simulink model "GridTiedInverterNew"  (R2024b)
settings: Solver=ode45  StartTime=0.0  StopTime=1  RelTol=1e-3
PreLoadFcn:
  | run('constants.m');
InitFcn:
  | run('constants.m');
values from neighbouring files (symbols this model uses):
  f_grid = 50    [constants.m]
  K_lqi = lqi(sys, Q_lqi, R)    [constants.m]
  K_lqr = lqr(sys, Q_lqr, R)    [constants.m]
  Ki = alpha * w_grid * w_grid * T_p * L_t / K_cm    (= 6152.69773705)    [constants.m]
  Ki_ = 10    [constants.m]
  Kp = (T_p * L_t * (2 * zeta * w_grid * alpha + w_grid * w_grid) - R_t) / K_cm    (= 28.1407059403)    [constants.m]
  Kp_ = 7000    [constants.m]
  L_t = 5e-2    (= 0.05)    [constants.m]
  P_rated_transformer = 10e3    (= 10000)    [constants.m]
  R_t = 0.15    [constants.m]
  t_breaker_on = 0.2    [constants.m]
  t_sample = 1 / f_sample    (= 1e-05)    [constants.m]
  V_dc = 300    [constants.m]
  V_grid = 230 * 4    (= 920)    [constants.m]
  V_t = 230    [constants.m]
undefined symbols (not defined in the file or in its folder): Kcp
libraries: spsIGBTDiodeLib x6, spsThreePhaseVIMeasurementLib x2, spsabctodq0Lib x2, spsPower3phInstantaneousLib x2, spsThreePhaseBreakerLib x1, spsThreePhaseSourceLib x1, spsPLL3phLib x1, spsThreePhaseSeriesRLCBranchLib x1, spsSawtoothGeneratorLib x1, spsTHDLib x1, SignalEditorBlockLib x1, eePwmGeneratorTwoLevel x1
settings Model: Creator=Gilbert  LastModifiedBy=Gilbert

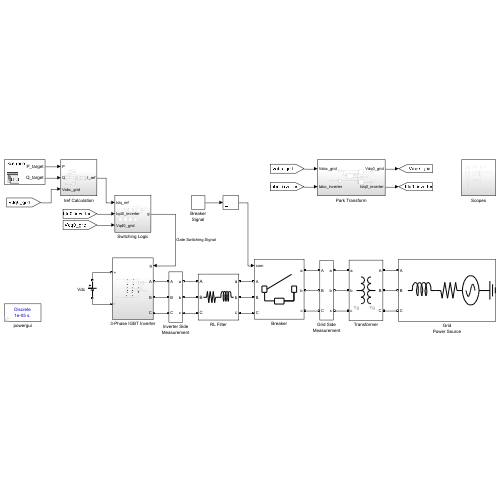
[thumbnail: Simulink's stored preview of the top-level diagram]
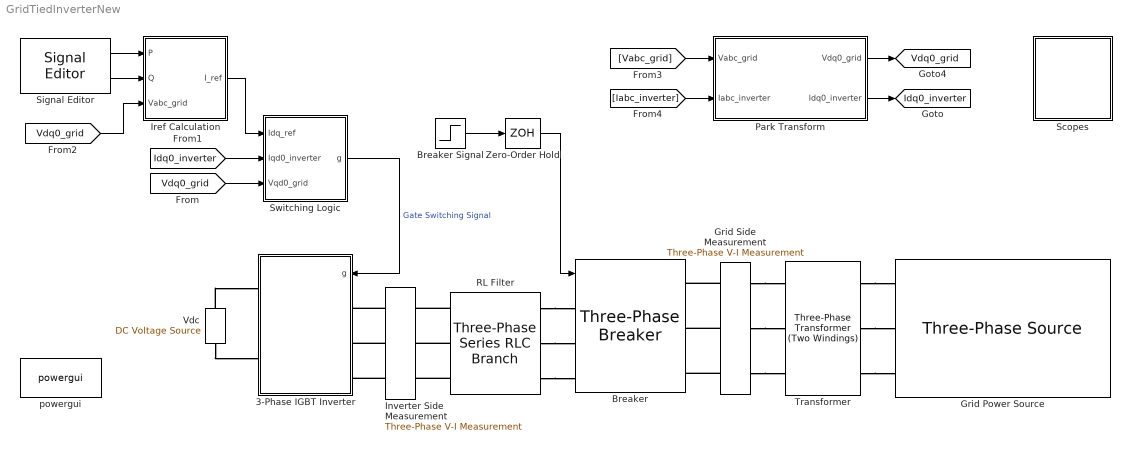
== system GridTiedInverterNew ==
  3-Phase IGBT Inverter : Subsystem
      settings: PortSchema="{\"entries\":[{\"content\":{\"sides\":[{\"content\":{\"connectorIds\":[\"LConn1\",\"LConn2\"]},\"type\":\"ConnectorPlacement.EquallySpacedRectSide\",\"uuid\":\"b894f77a-afb6-49ea-9e82-1d7302d1b564\"},{\"content\":{\"connectorIds\":[\"In1\",\"RConn1\",\"RConn2\",\"RConn3\"],\"side\":\"RIGHT\"},\"type\":\"ConnectorPlacement.EquallySpacedRectSide\",\"uuid\":\"2e0b49ec-be7c-4f2f-9d64-b0056ee6a69f\"},{\"content\":{\"side\":\"TOP\"},\"type\":\"ConnectorPlacement.EquallySpacedRectSide\",\"uuid\":\"c0a39988-5ea5-41cc-9f2f-ca3dfeeba5dd\"}]},\"type\":\"ConnectorPlacement.EquallySpacedConnector\",\"uuid\":\"873a7b17-3bf6-43e0-93b3-692e6d4c547a\"}],\"packageUris\":[\"http://schema.mathworks.com/mf0/Connector/R2020b\"],\"version\":\"1.0\"}"
  Breaker : spsThreePhaseBreakerLib/Three-Phase Breaker  InitialState=open  SwitchA=on  SwitchB=on  SwitchC=on  SwitchTimes="[1/60  5/60]"  External=on  BreakerResistance=0.01  SnubberResistance=1e6  SnubberCapacitance=inf  Measurements=None
  Breaker Signal : Step  Time=t_breaker_on  SampleTime=0
  Grid Power Source : spsThreePhaseSourceLib/Three-Phase Source  InternalConnection=Yg  VoltagePhases=off  Voltage=V_grid  PhaseAngle=phi_grid  Voltage_phases=[25e3 25e3 25e3]/sqrt(3)  PhaseAngles_phases=[0 -120 +120]  Frequency=f_grid  NonIdealSource=on  SpecifyImpedance=off  Resistance=0.8929e-12  Inductance=16.58e-12  ShortCircuitLevel=100e6  BaseVoltage=V_grid  XRratio=7  BusType=swing  Pref=10e3  Qref=0  Prefabc=[10e3, 10e3, 10e3]  Qrefabc=[0, 0, 0]  Qmin=-inf  Qmax=inf
  Grid Side Measurement : spsThreePhaseVIMeasurementLib/Three-Phase V-I Measurement  VoltageMeasurement=phase-to-phase  SetLabelV=on  LabelV=Vabc_grid  Vpu=off  VpuLL=off  CurrentMeasurement=yes  SetLabelI=on  LabelI=Iabc_grid  Ipu=off  Pbase=100e6  Vbase=500e3  OutputType=Complex  PhasorSimulation=off  PSBequivalent=0
  Inverter Side Measurement : spsThreePhaseVIMeasurementLib/Three-Phase V-I Measurement  VoltageMeasurement=phase-to-phase  SetLabelV=on  LabelV=Vabc_inverter  Vpu=off  VpuLL=off  CurrentMeasurement=yes  SetLabelI=on  LabelI=Iabc_inverter  Ipu=off  Pbase=100e6  Vbase=500e3  OutputType=Complex  PhasorSimulation=off  PSBequivalent=0
  Iref Calculation : Subsystem
  Park Transform : Subsystem
  RL Filter : spsThreePhaseSeriesRLCBranchLib/Three-Phase Series RLC Branch  LConnTagsString=A|B|C  RConnTagsString=A|B|C  BranchType=RL  Resistance=R_t  Inductance=L_t  Capacitance=1e-6  Measurements=None
  Scopes : Subsystem
  Signal Editor : SignalEditorBlockLib/Signal Editor  FileName=S_target_0.mat  ActiveScenario=Scenario  ActiveSignal=P_target  IsBus=off  OutputBusObjectStr=Bus: BusObject  SampleTime=0  Interpolate=off  ZeroCross=off  OutputAfterFinalValue=Holding final value  Unit=inherit  PreserveSignalName=on  ApplySigPropsToAllScenarios=on  ApplySigPropsToAllSignals=off
  Switching Logic : Subsystem
  Transformer : spsThreePhaseTransformerTwoWindingsLib/Three-Phase Transformer (Two Windings)  Winding1Connection=Yg  Winding2Connection=Yg  CoreType=Three single-phase transformers  SetSaturation=off  Hysteresis=off  DataFile='hysteresis'  SetInitialFlux=off  Measurements=None  UNITS=SI  NominalPower=[ P_rated_transformer , f_grid ]  Winding1=[V_grid 6.7712e-06 8.6214e-07]  Winding2=[V_t 4.232e-07 5.3883e-08]  Rm=1.6928  Lm=0.0053883  L0=5.3883e-06  Saturation=[0 0;532.5 2.8693;2.2187e+05 3.6344]  InitialFluxes=[1.9129 -1.9129 1.6737]  BreakLoop=off  DiscreteSolver=Trapezoidal iterative  DataType=on  TransfoNumber=1
  Vdc : spsDCVoltageSourceLib/DC Voltage Source  Amplitude=V_dc  Measurements=None
  Zero-Order Hold : ZeroOrderHold  SampleTime=t_sample
  powergui : sps_lib/powergui  Priority=1  SimulationMode=Discrete  SampleTime=t_sample  frequency=60  Iterations=50  frequencyindice=0  Pbase=100e6  ErrMax=1e-4  UnitsV=kV  UnitsW=MW  buscounter=0  FunctionMessages=off  echomessages=off  EnableUseOfTLC=off  CurrentSourceSwitches=off  DisableSnubberDevices=off  DisableRonSwitches=off  DisableVfSwitches=off  DisplayEquations=off  AutomaticDiscreteSolvers=off  SolverType=Tustin/Backward Euler (TBE)  Interpol=off  ExternalGateDelay=off  methode=off  Ts=100  x0status=blocks  SPID=on  SwTol=0  HookPort=off  NonlinearTolerance=1e-4  nMaxIteration=100  ContinueOnMaxIteration=off  RestoreLinks=warning  ResistiveCurrentMeasurement=off  Frange=[0:2:500]  Ylog=off  Xlog=on  ShowGrid=off  save=off  variable=ZData  structure=0  ZoomFFT=off  StartTime=0.0  cycles=1  DisplayStyle=1  fundamental=60  FreqAxis=off  MaxFrequency=1000  frequencyindicesteady=1  RmsSteady=1  display=off
  tag scope: Idq0_inverter=global, Vdq0_grid=global
  wires:
  [Vdq0_grid] -> Switching Logic/3(Vqd0_grid)
  [Vdq0_grid] -> Iref Calculation/3(Vabc_grid)
  Signal Editor/1 -> Iref Calculation/1(P)
  Signal Editor/2 -> Iref Calculation/2(Q)
  [Idq0_inverter] -> Switching Logic/2(Iqd0_inverter)
  Switching Logic/1(g) -> 3-Phase IGBT Inverter/1(g)  "Gate Switching Signal"
  Breaker Signal/1 -> Zero-Order Hold/1
  Zero-Order Hold/1 -> Breaker/1
  Iref Calculation/1(I_ref) -> Switching Logic/1(Idq_ref)
  Park Transform/2(Idq0_inverter) -> [Idq0_inverter]
  Park Transform/1(Vdq0_grid) -> [Vdq0_grid]
  [Vabc_grid] -> Park Transform/1(Vabc_grid)
  [Iabc_inverter] -> Park Transform/2(Iabc_inverter)
  connections:
  Transformer/LConn1 -- Grid Power Source/RConn1
  Transformer/LConn2 -- Grid Power Source/RConn2
  Transformer/LConn3 -- Grid Power Source/RConn3
  RL Filter/RConn1 -- Breaker/LConn1
  RL Filter/RConn2 -- Breaker/LConn2
  RL Filter/RConn3 -- Breaker/LConn3
  Grid Side Measurement/LConn1 -- Breaker/RConn1
  Grid Side Measurement/LConn2 -- Breaker/RConn2
  Grid Side Measurement/LConn3 -- Breaker/RConn3
  Vdc/LConn1 -- 3-Phase IGBT Inverter/LConn2
  Vdc/RConn1 -- 3-Phase IGBT Inverter/LConn1
  Inverter Side Measurement/LConn2 -- 3-Phase IGBT Inverter/RConn2
  Inverter Side Measurement/LConn3 -- 3-Phase IGBT Inverter/RConn3
  Inverter Side Measurement/LConn1 -- 3-Phase IGBT Inverter/RConn1
  Grid Side Measurement/RConn1 -- Transformer/RConn1
  Grid Side Measurement/RConn2 -- Transformer/RConn2
  Grid Side Measurement/RConn3 -- Transformer/RConn3
  RL Filter/LConn1 -- Inverter Side Measurement/RConn1
  RL Filter/LConn2 -- Inverter Side Measurement/RConn2
  RL Filter/LConn3 -- Inverter Side Measurement/RConn3

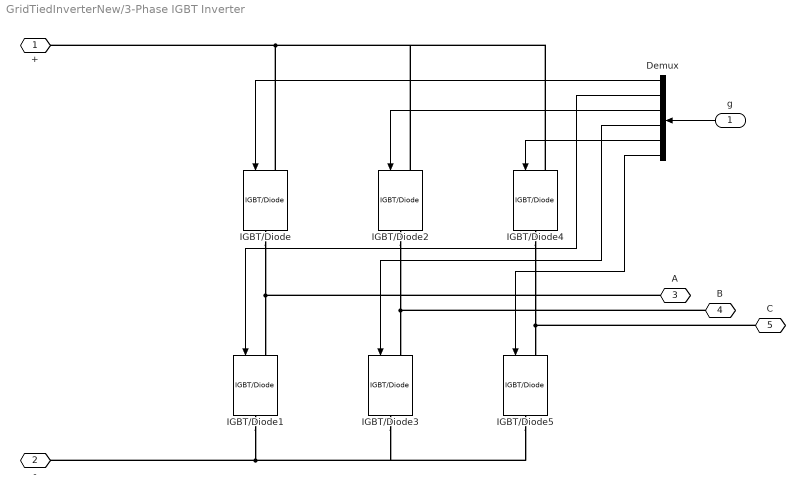
== system GridTiedInverterNew/3-Phase IGBT Inverter ==
  g : Inport
  Demux : Demux  Outputs=6
  IGBT/Diode{,1..5} (6 alike) : spsIGBTDiodeLib/IGBT//Diode  Ron=1e-3  Rs=1e5  Cs=inf  Measurements=off
  + : PMIOPort  Side=Left
  - : PMIOPort  Port=2  Side=Left
  A : PMIOPort  Port=3  Side=Right
  B : PMIOPort  Port=4  Side=Right
  C : PMIOPort  Port=5  Side=Right
  wires:
  Demux/3 -> IGBT/Diode2/1
  Demux/5 -> IGBT/Diode4/1
  Demux/2 -> IGBT/Diode1/1
  Demux/6 -> IGBT/Diode5/1
  Demux/4 -> IGBT/Diode3/1
  g/1 -> Demux/1
  Demux/1 -> IGBT/Diode/1
  connections:
  B/RConn1 -- IGBT/Diode3/LConn1 -- IGBT/Diode2/RConn1
  IGBT/Diode/LConn1 -- IGBT/Diode2/LConn1 -- IGBT/Diode4/LConn1 -- +/RConn1
  IGBT/Diode1/RConn1 -- IGBT/Diode5/RConn1 -- IGBT/Diode3/RConn1 -- -/RConn1
  A/RConn1 -- IGBT/Diode1/LConn1 -- IGBT/Diode/RConn1
  C/RConn1 -- IGBT/Diode5/LConn1 -- IGBT/Diode4/RConn1

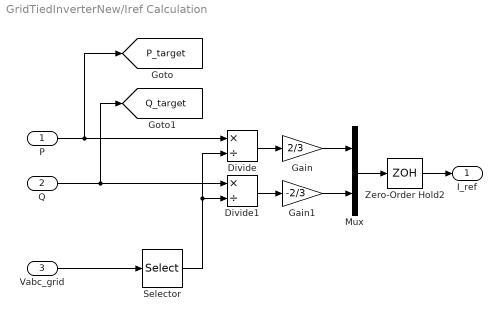
== system GridTiedInverterNew/Iref Calculation ==
  P : Inport
  Q : Inport  Port=2
  Vabc_grid : Inport  Port=3
  Divide : Product  Inputs=*/
  Divide1 : Product  Inputs=*/
  Gain : Gain  Gain=2/3
  Gain1 : Gain  Gain=-2/3
  Mux : Mux  Inputs=2
  Selector : Selector  InputPortWidth=3  IndexOptions=Index vector (dialog)  Indices=[1]  OutputSizes=1
  Zero-Order Hold2 : ZeroOrderHold  SampleTime=t_sample
  I_ref : Outport
  tag scope: P_target=global, Q_target=global
  wires:
  Vabc_grid/1 -> Selector/1
  P/1 -> [P_target], Divide/1
  Q/1 -> [Q_target], Divide1/1
  Mux/1 -> Zero-Order Hold2/1
  Selector/1 -> Divide/2, Divide1/2
  Divide/1 -> Gain/1
  Divide1/1 -> Gain1/1
  Gain/1 -> Mux/1
  Gain1/1 -> Mux/2
  Zero-Order Hold2/1 -> I_ref/1

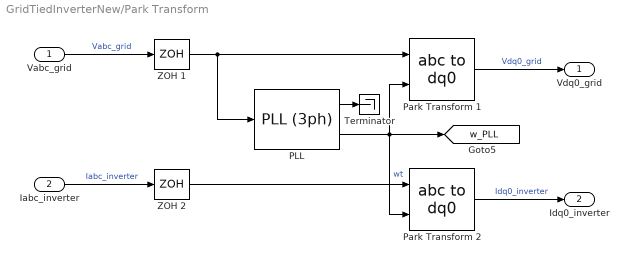
== system GridTiedInverterNew/Park Transform ==
  Vabc_grid : Inport
  Iabc_inverter : Inport  Port=2
  PLL : spsPLL3phLib/PLL (3ph)  Fmin=45  Par_Init=[0, f_grid]  ParK=[180, 3200, 1]  TcD=1e-4  MaxRateChangeFreq=12  FilterCutOffFreq=25  Ts=0  AGC=on
  Park Transform 1 : spsabctodq0Lib/abc to dq0  Alignment=90 degrees behind phase A axis
  Park Transform 2 : spsabctodq0Lib/abc to dq0  Alignment=90 degrees behind phase A axis
  Terminator : Terminator
  ZOH 1 : ZeroOrderHold  SampleTime=t_sample
  ZOH 2 : ZeroOrderHold  SampleTime=t_sample
  Vdq0_grid : Outport
  Idq0_inverter : Outport  Port=2
  tag scope: w_PLL=global
  wires:
  PLL/2 -> Park Transform 2/2, Park Transform 1/2, [w_PLL]  "wt"
  Vabc_grid/1 -> ZOH 1/1  "Vabc_grid"
  PLL/1 -> Terminator/1
  Iabc_inverter/1 -> ZOH 2/1  "Iabc_inverter"
  ZOH 1/1 -> PLL/1, Park Transform 1/1
  ZOH 2/1 -> Park Transform 2/1
  Park Transform 2/1 -> Idq0_inverter/1  "Idq0_inverter"
  Park Transform 1/1 -> Vdq0_grid/1  "Vdq0_grid"

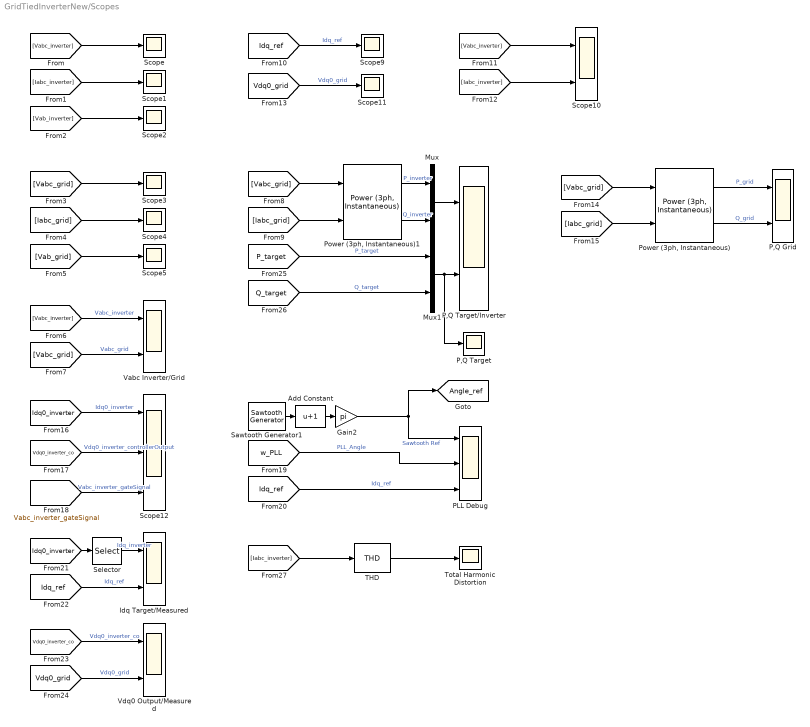
== system GridTiedInverterNew/Scopes ==
  Add Constant : Bias  Bias=1  SaturateOnIntegerOverflow=off
  Gain2 : Gain  Gain=pi
  Idq Target/Measured : Scope  NumInputPorts=2
  Mux : Mux  Inputs=2
  Mux1 : Mux  Inputs=2
  P,Q Grid : Scope  NumInputPorts=2
  P,Q Target : Scope
  P,Q Target/Inverter : Scope  NumInputPorts=2
  PLL Debug : Scope  NumInputPorts=3
  "Power (3ph, Instantaneous)" : spsPower3phInstantaneousLib/Power (3ph, Instantaneous)
  "Power (3ph, Instantaneous)1" : spsPower3phInstantaneousLib/Power (3ph, Instantaneous)
  Sawtooth Generator1 : spsSawtoothGeneratorLib/Sawtooth Generator  Freq=50  Phase=0  Ts=0
  Scope{,1..5,9,11} (8 alike) : Scope
  Scope10 : Scope  NumInputPorts=2
  Scope12 : Scope  NumInputPorts=3
  Selector : Selector  InputPortWidth=3  IndexOptions=Index vector (dialog)  Indices=[1 2]  OutputSizes=1
  THD : spsTHDLib/THD  Freq=f_grid  Ts=t_sample
  Total Harmonic Distortion : Scope
  Vabc Inverter/Grid : Scope  NumInputPorts=2
  Vdq0 Output/Measured : Scope  NumInputPorts=2
  tag scope: Angle_ref=global
  wires:
  [Vabc_inverter] -> Scope/1
  [Iabc_inverter] -> Scope1/1
  [Vab_inverter] -> Scope2/1
  [Vabc_grid] -> Scope3/1
  [Iabc_grid] -> Scope4/1
  [Vab_grid] -> Scope5/1
  [Vabc_inverter] -> Vabc Inverter/Grid/1  "Vabc_inverter"
  [Vabc_grid] -> Vabc Inverter/Grid/2  "Vabc_grid"
  [Vabc_grid] -> "Power (3ph, Instantaneous)1"/1
  [Iabc_grid] -> "Power (3ph, Instantaneous)1"/2
  "Power (3ph, Instantaneous)1"/1 -> Mux/1  "P_inverter"
  "Power (3ph, Instantaneous)1"/2 -> Mux/2  "Q_inverter"
  [Idq_ref] -> Scope9/1  "Idq_ref"
  [Vabc_inverter] -> Scope10/1
  [Iabc_inverter] -> Scope10/2
  [Vdq0_grid] -> Scope11/1  "Vdq0_grid"
  [Vabc_grid] -> "Power (3ph, Instantaneous)"/1
  [Iabc_grid] -> "Power (3ph, Instantaneous)"/2
  "Power (3ph, Instantaneous)"/1 -> P,Q Grid/1  "P_grid"
  "Power (3ph, Instantaneous)"/2 -> P,Q Grid/2  "Q_grid"
  [Idq0_inverter] -> Scope12/1  "Idq0_inverter"
  [Vdq0_inverter_co] -> Scope12/2  "Vdq0_inverter_controllerOutput"
  [Vabc_inverter_gateSignal] -> Scope12/3  "Vabc_inverter_gateSignal"
  Add Constant/1 -> Gain2/1
  Sawtooth Generator1/1 -> Add Constant/1
  [w_PLL] -> PLL Debug/2  "PLL_Angle"
  [Idq_ref] -> PLL Debug/3  "Idq_ref"
  Gain2/1 -> [Angle_ref], PLL Debug/1  "Sawtooth Ref"
  [Idq0_inverter] -> Selector/1
  [Idq_ref] -> Idq Target/Measured/2  "Idq_ref"
  [Vdq0_grid] -> Vdq0 Output/Measured/2  "Vdq0_grid"
  [Vdq0_inverter_co] -> Vdq0 Output/Measured/1  "Vdq0_inverter_co"
  [P_target] -> Mux1/1  "P_target"
  [Q_target] -> Mux1/2  "Q_target"
  Mux/1 -> P,Q Target/Inverter/1
  Mux1/1 -> P,Q Target/Inverter/2, P,Q Target/1
  [Iabc_inverter] -> THD/1
  THD/1 -> Total Harmonic Distortion/1
  Selector/1 -> Idq Target/Measured/1  "Idq_inverter"

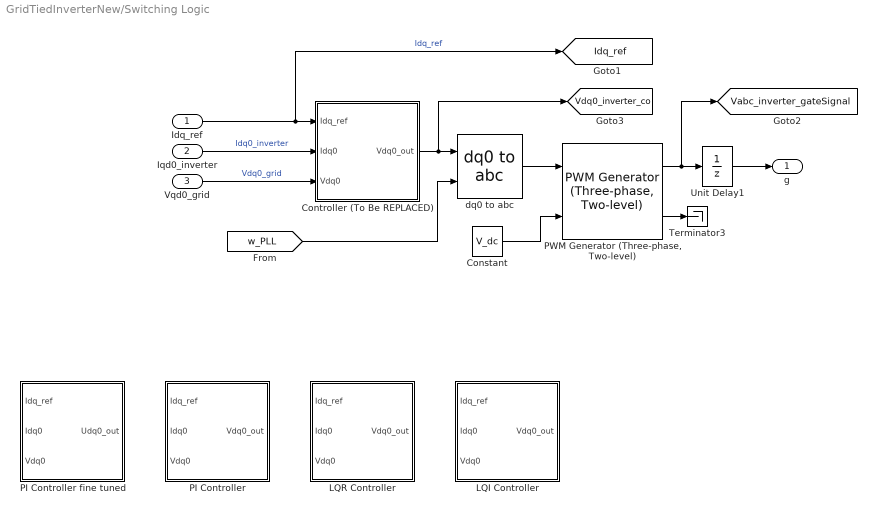
== system GridTiedInverterNew/Switching Logic ==
  Idq_ref : Inport
  Iqd0_inverter : Inport  Port=2
  Vqd0_grid : Inport  Port=3
  Constant : Constant  Value=V_dc
  Controller (To Be REPLACED) : Subsystem
  LQI Controller : Subsystem
  LQR Controller : Subsystem
  PI Controller : Subsystem
  PI Controller fine tuned : Subsystem
  "PWM Generator (Three-phase, Two-level)" : eePwmGeneratorTwoLevel/PWM Generator (Three-phase, Two-level)  PWMMode=Continuous PWM (CPWM)  CPWMMode=SVM: space vector modulation  DPWMMode=60 DPWM: 60 degree discontinuous PWM  fsw=f_sw  Ts=t_sample
      settings: LibrarySourceBlock=|
      | ee_sl_lib/Pulse Width
      | Modulation/PWM Generator
      | (Three-phase, Two-level)
  Terminator3 : Terminator
  Unit Delay1 : UnitDelay  SampleTime=t_sample  HasFrameUpgradeWarning=on
  dq0 to abc : spsdq0toabcLib/dq0 to abc  Alignment=90 degrees behind phase A axis
  g : Outport
  tag scope: Idq_ref=global, Vabc_inverter_gateSignal=global, Vdq0_inverter_co=global
  wires:
  "PWM Generator (Three-phase, Two-level)"/1 -> [Vabc_inverter_gateSignal], Unit Delay1/1
  Unit Delay1/1 -> g/1
  Constant/1 -> "PWM Generator (Three-phase, Two-level)"/2
  "PWM Generator (Three-phase, Two-level)"/2 -> Terminator3/1
  dq0 to abc/1 -> "PWM Generator (Three-phase, Two-level)"/1
  Vqd0_grid/1 -> Controller (To Be REPLACED)/3(Vdq0)  "Vdq0_grid"
  Iqd0_inverter/1 -> Controller (To Be REPLACED)/2(Idq0)  "Idq0_inverter"
  Controller (To Be REPLACED)/1(Vdq0_out) -> dq0 to abc/1, [Vdq0_inverter_co]
  Idq_ref/1 -> Controller (To Be REPLACED)/1(Idq_ref), [Idq_ref]  "Idq_ref"
  [w_PLL] -> dq0 to abc/2

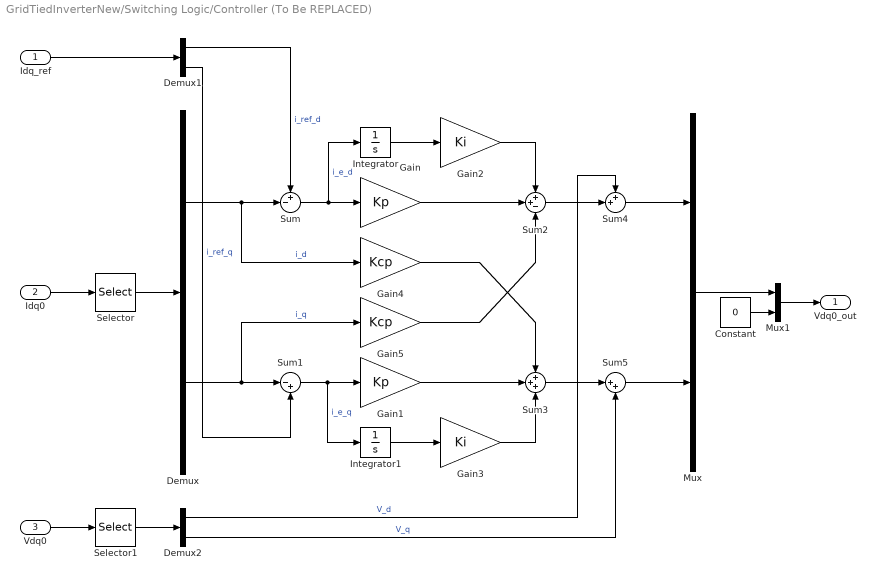
== system GridTiedInverterNew/Switching Logic/Controller (To Be REPLACED) ==
  Idq_ref : Inport
  Idq0 : Inport  Port=2
  Vdq0 : Inport  Port=3
  Constant : Constant  Value=0
  Demux : Demux  Outputs=2
  Demux1 : Demux  Outputs=2
  Demux2 : Demux  Outputs=2
  Gain : Gain  Gain=Kp
  Gain1 : Gain  Gain=Kp
  Gain2 : Gain  Gain=Ki
  Gain3 : Gain  Gain=Ki
  Gain4 : Gain  Gain=Kcp
  Gain5 : Gain  Gain=Kcp
  Integrator : Integrator
  Integrator1 : Integrator
  Mux : Mux  Inputs=2
  Mux1 : Mux  Inputs=2
  Selector : Selector  InputPortWidth=3  IndexOptions=Index vector (dialog)  Indices=[1 2]  OutputSizes=1
  Selector1 : Selector  InputPortWidth=3  IndexOptions=Index vector (dialog)  Indices=[1 2]  OutputSizes=1
  Sum : Sum  Inputs=+-|
  Sum1 : Sum  Inputs=|-+
  Sum2 : Sum  Inputs=++-
  Sum3 : Sum  Inputs=+++
  Sum4 : Sum  Inputs=++|
  Sum5 : Sum  Inputs=|++
  Vdq0_out : Outport
  wires:
  Gain5/1 -> Sum2/3
  Gain4/1 -> Sum3/1
  Demux2/2 -> Sum5/2  "V_q"
  Demux2/1 -> Sum4/1  "V_d"
  Sum5/1 -> Mux/2
  Sum3/1 -> Sum5/1
  Sum4/1 -> Mux/1
  Sum2/1 -> Sum4/2
  Selector1/1 -> Demux2/1
  Vdq0/1 -> Selector1/1
  Gain3/1 -> Sum3/3
  Integrator1/1 -> Gain3/1
  Gain1/1 -> Sum3/2
  Gain2/1 -> Sum2/1
  Integrator/1 -> Gain2/1
  Gain/1 -> Sum2/2
  Sum/1 -> Gain/1, Integrator/1  "i_e_d"
  Mux1/1 -> Vdq0_out/1
  Constant/1 -> Mux1/2
  Mux/1 -> Mux1/1
  Selector/1 -> Demux/1
  Idq0/1 -> Selector/1
  Sum1/1 -> Integrator1/1, Gain1/1  "i_e_q"
  Demux1/2 -> Sum1/2  "i_ref_q"
  Demux/2 -> Sum1/1, Gain5/1  "i_q"
  Demux1/1 -> Sum/1  "i_ref_d"
  Demux/1 -> Sum/2, Gain4/1  "i_d"
  Idq_ref/1 -> Demux1/1

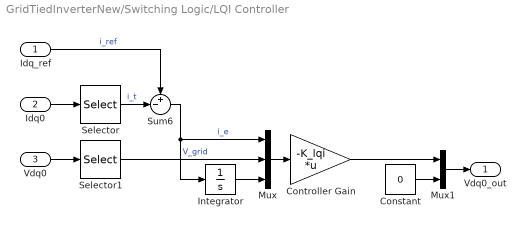
== system GridTiedInverterNew/Switching Logic/LQI Controller ==
  Idq_ref : Inport
  Idq0 : Inport  Port=2
  Vdq0 : Inport  Port=3
  " Integrator " : Integrator
  Constant : Constant  Value=0
  Controller Gain : Gain  Gain=-K_lqi  Multiplication=Matrix(K*u)
  Mux : Mux  Inputs=3
  Mux1 : Mux  Inputs=2
  Selector : Selector  InputPortWidth=3  IndexOptions=Index vector (dialog)  Indices=[1 2]  OutputSizes=1
  Selector1 : Selector  InputPortWidth=3  IndexOptions=Index vector (dialog)  Indices=[1 2]  OutputSizes=1
  Sum6 : Sum  Inputs=+-|
  Vdq0_out : Outport
  wires:
  Selector1/1 -> Mux/2  "V_grid"
  Vdq0/1 -> Selector1/1
  Idq0/1 -> Selector/1
  Idq_ref/1 -> Sum6/1  "i_ref"
  Selector/1 -> Sum6/2  "i_t"
  Sum6/1 -> " Integrator "/1, Mux/1  "i_e"
  Constant/1 -> Mux1/2
  Mux1/1 -> Vdq0_out/1
  Controller Gain/1 -> Mux1/1
  Mux/1 -> Controller Gain/1
  " Integrator "/1 -> Mux/3

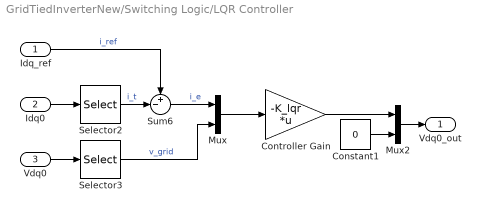
== system GridTiedInverterNew/Switching Logic/LQR Controller ==
  Idq_ref : Inport
  Idq0 : Inport  Port=2
  Vdq0 : Inport  Port=3
  Constant1 : Constant  Value=0
  Controller Gain : Gain  Gain=-K_lqr  Multiplication=Matrix(K*u)
  Mux : Mux  Inputs=2
  Mux2 : Mux  Inputs=2
  Selector2 : Selector  InputPortWidth=3  IndexOptions=Index vector (dialog)  Indices=[1 2]  OutputSizes=1
  Selector3 : Selector  InputPortWidth=3  IndexOptions=Index vector (dialog)  Indices=[1 2]  OutputSizes=1
  Sum6 : Sum  Inputs=+-|
  Vdq0_out : Outport
  wires:
  Mux2/1 -> Vdq0_out/1
  Constant1/1 -> Mux2/2
  Selector2/1 -> Sum6/2  "i_t"
  Sum6/1 -> Mux/1  "i_e"
  Idq_ref/1 -> Sum6/1  "i_ref"
  Selector3/1 -> Mux/2  "v_grid"
  Idq0/1 -> Selector2/1
  Vdq0/1 -> Selector3/1
  Controller Gain/1 -> Mux2/1
  Mux/1 -> Controller Gain/1

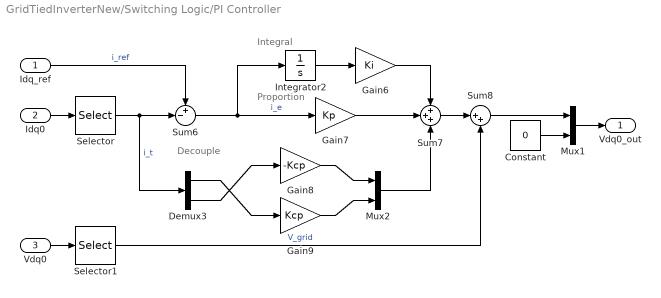
== system GridTiedInverterNew/Switching Logic/PI Controller ==
  note: Proportion
  note: Decouple
  note: Integral
  Idq_ref : Inport
  Idq0 : Inport  Port=2
  Vdq0 : Inport  Port=3
  Constant : Constant  Value=0
  Demux3 : Demux  Outputs=2
  Gain6 : Gain  Gain=Ki
  Gain7 : Gain  Gain=Kp
  Gain8 : Gain  Gain=-Kcp
  Gain9 : Gain  Gain=Kcp
  Integrator2 : Integrator
  Mux1 : Mux  Inputs=2
  Mux2 : Mux  Inputs=2
  Selector : Selector  InputPortWidth=3  IndexOptions=Index vector (dialog)  Indices=[1 2]  OutputSizes=1
  Selector1 : Selector  InputPortWidth=3  IndexOptions=Index vector (dialog)  Indices=[1 2]  OutputSizes=1
  Sum6 : Sum  Inputs=+-|
  Sum7 : Sum  Inputs=+++
  Sum8 : Sum  Inputs=|++
  Vdq0_out : Outport
  wires:
  Idq0/1 -> Selector/1
  Constant/1 -> Mux1/2
  Mux1/1 -> Vdq0_out/1
  Vdq0/1 -> Selector1/1
  Idq_ref/1 -> Sum6/1  "i_ref"
  Selector/1 -> Demux3/1, Sum6/2  "i_t"
  Sum6/1 -> Integrator2/1, Gain7/1  "i_e"
  Demux3/1 -> Gain9/1
  Integrator2/1 -> Gain6/1
  Demux3/2 -> Gain8/1
  Gain9/1 -> Mux2/2
  Gain8/1 -> Mux2/1
  Gain7/1 -> Sum7/2
  Gain6/1 -> Sum7/1
  Sum7/1 -> Sum8/1
  Selector1/1 -> Sum8/2  "V_grid"
  Sum8/1 -> Mux1/1
  Mux2/1 -> Sum7/3

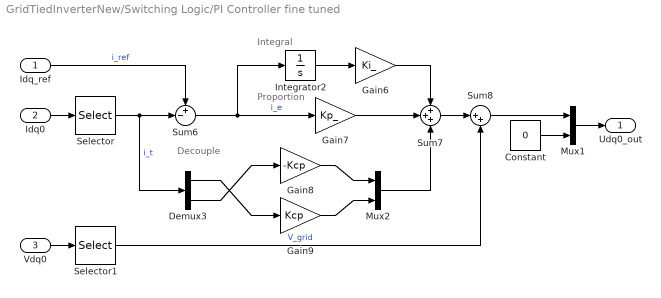
== system GridTiedInverterNew/Switching Logic/PI Controller fine tuned ==
  note: Integral
  note: Decouple
  note: Proportion
  Idq_ref : Inport
  Idq0 : Inport  Port=2
  Vdq0 : Inport  Port=3
  Constant : Constant  Value=0
  Demux3 : Demux  Outputs=2
  Gain6 : Gain  Gain=Ki_
  Gain7 : Gain  Gain=Kp_
  Gain8 : Gain  Gain=-Kcp
  Gain9 : Gain  Gain=Kcp
  Integrator2 : Integrator
  Mux1 : Mux  Inputs=2
  Mux2 : Mux  Inputs=2
  Selector : Selector  InputPortWidth=3  IndexOptions=Index vector (dialog)  Indices=[1 2]  OutputSizes=1
  Selector1 : Selector  InputPortWidth=3  IndexOptions=Index vector (dialog)  Indices=[1 2]  OutputSizes=1
  Sum6 : Sum  Inputs=+-|
  Sum7 : Sum  Inputs=+++
  Sum8 : Sum  Inputs=|++
  Udq0_out : Outport
  wires:
  Mux2/1 -> Sum7/3
  Sum8/1 -> Mux1/1
  Selector1/1 -> Sum8/2  "V_grid"
  Sum7/1 -> Sum8/1
  Gain6/1 -> Sum7/1
  Gain7/1 -> Sum7/2
  Gain8/1 -> Mux2/1
  Gain9/1 -> Mux2/2
  Demux3/2 -> Gain8/1
  Integrator2/1 -> Gain6/1
  Demux3/1 -> Gain9/1
  Sum6/1 -> Gain7/1, Integrator2/1  "i_e"
  Selector/1 -> Sum6/2, Demux3/1  "i_t"
  Idq_ref/1 -> Sum6/1  "i_ref"
  Vdq0/1 -> Selector1/1
  Mux1/1 -> Udq0_out/1
  Constant/1 -> Mux1/2
  Idq0/1 -> Selector/1
